simulink model "noninverting1"  (R2020b)
settings: Solver=VariableStepAuto  StartTime=0.0  StopTime=0.2  MaxStep=0.00002  RelTol=1e-3  AbsTol=1e-3  EnableMultiTasking=on
libraries: fl_lib x8, nesl_utility x3
CloseFcn:
  | try,close(h1_ssc_opamp_noninverting),end
  | clear simlog_ssc_opamp_noninverting
Description:
  | Op-Amp Circuit - Noninverting Amplifier
settings Model: Creator=The MathWorks, Inc.  LastModifiedBy=bolic
settings SolverCC: AutoScaleAbsTol=off
settings DataIOCC: LimitDataPoints=on  SaveFormat=Array  ReturnWorkspaceOutputs=off
settings OptimizationCC: LifeSpan=inf
settings DebuggingCC: SolverPrmCheckMsg=warning  AllowSymbolicDim=off  PregeneratedLibrarySubsystemCodeDiagnostic=none  SFUnexpectedBacktrackingDiag=warning  SFNoUnconditionalDefaultTransitionDiag=warning  SFExecutionAtInitializationDiag=none  ArithmeticOperatorsInVariantConditions=warning
settings HardwareCC: ProdBitPerPointer=32  ProdBitPerSizeT=32  ProdBitPerPtrDiffT=32  ProdLargestAtomicFloat=None  ProdIntDivRoundTo=Undefined  ProdEndianess=Unspecified  ProdWordSize=32  ProdHWDeviceType=32-bit Generic
settings ModelReferenceCC: PropagateSignalLabelsOutOfModel=off
settings SFSimCC: SimUseLocalCustomCode=off  CustomCodeUndefinedFunction=UseInterfaceOnly
settings RTWCC: RTWUseLocalCustomCode=off
settings CodeAppCC: StateflowObjectComments=on
settings GRTTargetCC: TargetLangStandard=C89/C90 (ANSI)
settings ConfigComp: CovMetricSettings=dw  CovSaveCumulativeToWorkspaceVar=on  CovSaveSingleToWorkspaceVar=on  CovExternalEMLEnable=off  CovSFcnEnable=off
settings SimscapeCC: SimscapeLogType=all  SimscapeLogSimulationStatistics=on  SimscapeLogName=simlog_ssc_opamp_noninverting  SimscapeLogDataHistory=10000

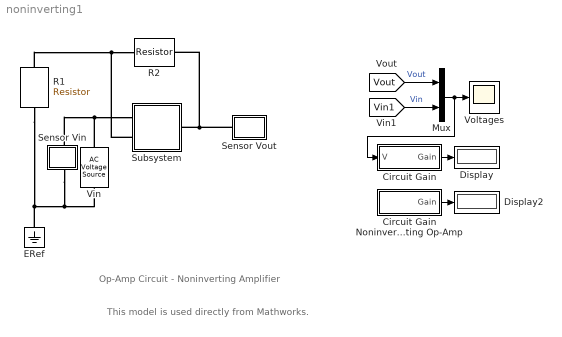
== system noninverting1 ==
  note: Op-Amp Circuit - Noninverting Amplifier
  note: This model is used directly from Mathworks.
  Circuit Gain : Subsystem
  Circuit Gain Noninverting Op-Amp : Subsystem
      mask init:
      | set_param([gcb '/R1'],'Value',...
      |     get_param([bdroot '/R1'],'r'));
      | set_param([gcb '/R2'],'Value',...
      |     get_param([bdroot '/R2'],'r'));
      mask Display: disp('1+R2/R1')
  Display : Display
  Display2 : Display
  ERef : fl_lib/Electrical/Electrical Elements/Electrical Reference
      settings: SourceProductName=Foundation Library
  Mux : Mux  Inputs=2
  R1 : fl_lib/Electrical/Electrical Elements/Resistor  R=1 kOhm  i_specify=off  i_priority=High  i=0 A  i_nominal_specify=off  i_nominal_unit=A  i_nominal_value=1  v_specify=off  v_priority=High  v=0 V  v_nominal_specify=off  v_nominal_unit=V  v_nominal_value=1
      settings: AttributesFormatString=%<R> %<R_unit>  SourceProductName=Foundation Library
  R2 : fl_lib/Electrical/Electrical Elements/Resistor  R=10 kOhm  i_specify=off  i_priority=High  i=0 A  i_nominal_specify=off  i_nominal_unit=A  i_nominal_value=1  v_specify=off  v_priority=High  v=0 V  v_nominal_specify=off  v_nominal_unit=V  v_nominal_value=1
      settings: AttributesFormatString=%<R> %<R_unit>  SourceProductName=Foundation Library
  Sensor Vin : Subsystem
      settings: PortSchema="{\"entries\":[{\"content\":{\"sides\":[{\"content\":{\"connectorIds\":[]},\"type\":\"ConnectorPlacement.EquallySpacedRectSide\",\"uuid\":\"180edbd0-ff9a-4c2a-b7ea-01c6495ef3f4\"},{\"content\":{\"connectorIds\":[],\"side\":\"RIGHT\"},\"type\":\"ConnectorPlacement.EquallySpacedRectSide\",\"uuid\":\"2a3a3e73-0f6e-4fdb-90f8-40639a57a771\"},{\"content\":{\"connectorIds\":[\"LConn1\"],\"side\":\"TOP\"},\"type\":\"ConnectorPlacement.EquallySpacedRectSide\",\"uuid\":\"aea7ede2-6342-4686-90e1-8fdbf5b2ff13\"},{\"content\":{\"connectorIds\":[\"RConn1\"],\"side\":\"BOTTOM\"},\"type\":\"ConnectorPlacement.EquallySpacedRectSide\",\"uuid\":\"69a303fe-98b8-4050-8c6a-e3ba1d8c5387\"},{\"content\":{\"connectorIds\":[],\"side\":\"HIDDEN\"},\"type\":\"ConnectorPlacement.EquallySpacedRectSide\",\"uuid\":\"ab147681-5eb0-41fe-980d-a1974a4dacaf\"}]},\"type\":\"ConnectorPlacement.EquallySpacedConnector\",\"uuid\":\"f20915ef-6c1b-4295-9fb9-8cacf4f1b712\"}],\"packageUris\":[\"http://schema.mathworks.com/mf0/Connector/R2020b\"],\"version\":\"1.0\"}"
      mask Display: disp('Vin')
  Sensor Vout : Subsystem
      mask Display: disp('Vo')
  Subsystem : Subsystem
      mask Display: image('op_amp.png')
  Vin : fl_lib/Electrical/Electrical Sources/AC Voltage Source  amp=0.1 V  shift=0 deg  frequency=10 Hz  omega=0 rad/s
      settings: SourceProductName=Foundation Library
  Voltages : Scope
  wires:
  Mux/1 -> Circuit Gain/1(V), Voltages/1
  [Vout] -> Mux/1  "Vout"
  [Vin1] -> Mux/2  "Vin"
  Circuit Gain/1(Gain) -> Display/1
  Circuit Gain Noninverting Op-Amp/1(Gain) -> Display2/1
  connections:
  Sensor Vout/LConn1 -- R2/LConn1 -- Subsystem/RConn1
  R1/LConn1 -- Subsystem/LConn2 -- R2/RConn1
  R1/RConn1 -- Vin/RConn1 -- Sensor Vin/RConn1 -- ERef/LConn1
  Vin/LConn1 -- Sensor Vin/LConn1 -- Subsystem/LConn1

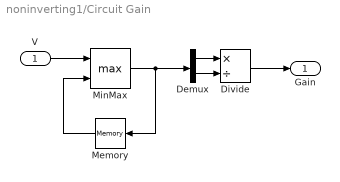
== system noninverting1/Circuit Gain ==
  V : Inport
  Demux : Demux  Outputs=2
  Divide : Product  Inputs=*/
  Memory : Memory  InitialCondition=1e-15  InheritSampleTime=on
  MinMax : MinMax  DisableCoverage=on  Function=max  Inputs=2  OutDataTypeStr=Inherit: Inherit via back propagation  ZeroCross=off
      settings: LockScale=on
  Gain : Outport  VectorParamsAs1DForOutWhenUnconnected=off
  wires:
  Divide/1 -> Gain/1
  Demux/2 -> Divide/2
  Memory/1 -> MinMax/2
  MinMax/1 -> Demux/1, Memory/1
  Demux/1 -> Divide/1
  V/1 -> MinMax/1

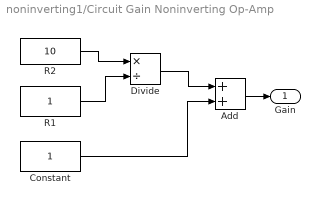
== system noninverting1/Circuit Gain Noninverting Op-Amp ==
  Add : Sum
  Constant : Constant
  Divide : Product  Inputs=*/
  R1 : Constant
  R2 : Constant  Value=10
  Gain : Outport  VectorParamsAs1DForOutWhenUnconnected=off
  wires:
  R2/1 -> Divide/1
  R1/1 -> Divide/2
  Add/1 -> Gain/1
  Divide/1 -> Add/1
  Constant/1 -> Add/2

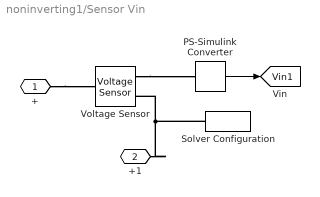
== system noninverting1/Sensor Vin ==
  PS-Simulink Converter : nesl_utility/PS-Simulink Converter  PhysicalDomain=network_engine_domain  SubClassName=ps_output  LeftPortType=input  RightPortType=output  PseudoPeriodic=off  Frequencies=[]  Unit=1  AffineConversion=off
      settings: SourceProductName=Utilities
  Solver Configuration : nesl_utility/Solver Configuration  PhysicalDomain=network_engine_domain  SubClassName=solver  LeftPortType=input  RightPortType=generic  Tones=[]  Harmonics=[]  SimulateNoise=off  Profile=off  UseLocalSampling=off  EnableSwitchedLinearOptims=on  FrequencyDomain=off  UseCCode=off  RelTol=0.001  AbsTol=1e-06  MinStep=1e-09  ToWorkspace=off  RevertToSquareIcSolve=off  NumHomotopyIterations=100  PhasorMode=off  PhasorModeNumHarmonics=1  DoDC=off  ResidualTolerance=1e-9  UseLocalSolver=off  LocalSolverChoice=NE_BACKWARD_EULER_ADVANCER  LocalSolverSampleTime=1e-6  DoFixedCost=off  MaxNonlinIter=3  MaxModeIter=2  ComputeImpulses=off  ImpulseIterations=2  LinearAlgebra=auto  EquationFormulation=NE_TIME_EF  DelaysMemoryBudget=1024  AutomaticFiltering=on  FilteringTimeConstant=0.001  PartitionStorageMethod=AS_NEEDED  PartitionMemoryBudget=1024  PartitionMethod=FAST
      settings: SourceProductName=Utilities
  Voltage Sensor : fl_lib/Electrical/Electrical Sensors/Voltage Sensor
      settings: SourceProductName=Foundation Library
  + : PMIOPort  Side=Left
  +1 : PMIOPort  Port=2  Side=Right
  tag scope: Vin1=global
  wires:
  PS-Simulink Converter/1 -> [Vin1]
  connections:
  +/RConn1 -- Voltage Sensor/LConn1
  Voltage Sensor/RConn1 -- PS-Simulink Converter/LConn1
  Solver Configuration/RConn1 -- +1/RConn1 -- Voltage Sensor/RConn2

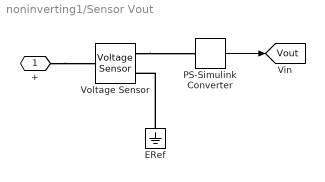
== system noninverting1/Sensor Vout ==
  ERef : fl_lib/Electrical/Electrical Elements/Electrical Reference
      settings: SourceProductName=Foundation Library
  PS-Simulink Converter : nesl_utility/PS-Simulink Converter  PhysicalDomain=network_engine_domain  SubClassName=ps_output  LeftPortType=input  RightPortType=output  PseudoPeriodic=off  Frequencies=[]  Unit=1  AffineConversion=off
      settings: SourceProductName=Utilities
  Voltage Sensor : fl_lib/Electrical/Electrical Sensors/Voltage Sensor
      settings: SourceProductName=Foundation Library
  + : PMIOPort  Side=Left
  tag scope: Vout=global
  wires:
  PS-Simulink Converter/1 -> [Vout]
  connections:
  ERef/LConn1 -- Voltage Sensor/RConn2
  Voltage Sensor/RConn1 -- PS-Simulink Converter/LConn1
  +/RConn1 -- Voltage Sensor/LConn1

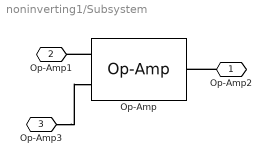
== system noninverting1/Subsystem ==
  Op-Amp : fl_lib/Electrical/Electrical Elements/Op-Amp  outI_specify=off  outI_priority=High  outI=0 A  outI_nominal_specify=off  outI_nominal_unit=A  outI_nominal_value=1
      settings: SourceProductName=Foundation Library
  Op-Amp2 : PMIOPort  Side=Right
  Op-Amp1 : PMIOPort  Port=2  Side=Left
  Op-Amp3 : PMIOPort  Port=3  Side=Left
  connections:
  Op-Amp3/RConn1 -- Op-Amp/LConn1
  Op-Amp2/RConn1 -- Op-Amp/RConn1
  Op-Amp/LConn2 -- Op-Amp1/RConn1
